simulink model "OneCombinedLQR"  (R2025b)
settings: Solver=ode4  StartTime=0.0  StopTime=T_end  FixedStep=0.001  RelTol=1e-3
values from neighbouring files (symbols this model uses):
  h_ref = double(h_ref)    [main.m]
  K_lqr = double(K_lqr)    [main.m]
  P = [x_ref y_ref]    [main.m]
  S_path = [S_path; S_raw(end)]    [main.m]
  theta_ref_unwrapped = unwrap(theta_ref)    [main.m]
  vd_path = min(vd_path, vd_max)    [main.m]
  wd_path = max(min(wd_path, wd_max), -wd_max)    [main.m]
  x_init = [phi_h; 0; theta_h; 0; v_h; omega_h; x_h; y_h]    [main.m]
settings Model: Creator=mwali  LastModifiedBy=mwali

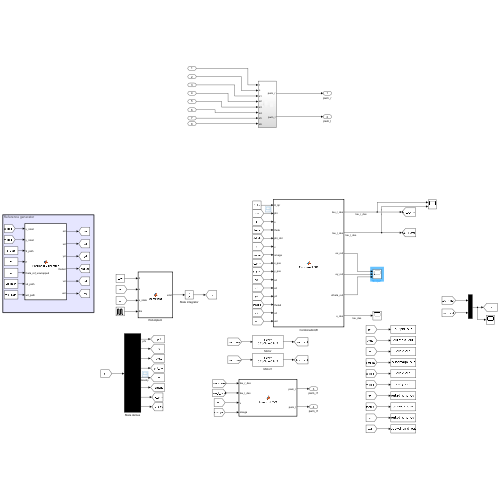
[thumbnail: Simulink's stored preview of the top-level diagram]
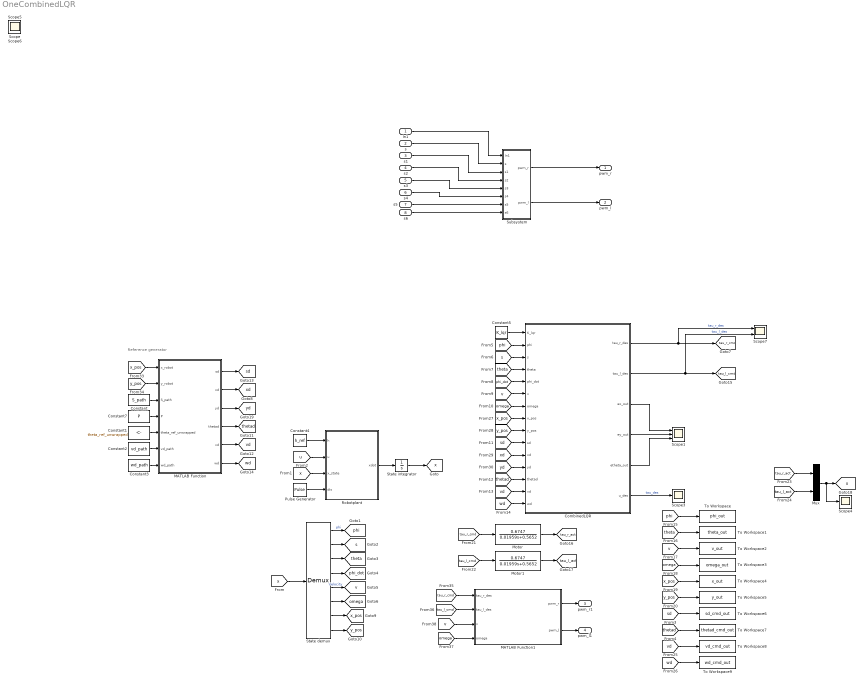
== system OneCombinedLQR ==
  note: Reference generator
  In1 : Inport
  s : Inport  Port=2
  s1 : Inport  Port=3
  s2 : Inport  Port=4
  s3 : Inport  Port=5
  s4 : Inport  Port=6
  s5 : Inport  Port=7
  s6 : Inport  Port=8
  CombinedLQR : MATLAB Function  TreatAsAtomicUnit=on
  Constant : Constant  Value=S_path
  Constant1 : Constant  Value=theta_ref_unwrapped
  Constant2 : Constant  Value=vd_path
  Constant3 : Constant  Value=wd_path
  Constant4 : Constant  Value=h_ref
  Constant5 : Constant  Value=K_lqr
  Constant7 : Constant  Value=P
  MATLAB Function : MATLAB Function  TreatAsAtomicUnit=on
  MATLAB Function1 : MATLAB Function  TreatAsAtomicUnit=on
  Motor : TransferFcn  Numerator=[0.6747]  Denominator=[0.01959 0.5652]
  Motor1 : TransferFcn  Numerator=[0.6747]  Denominator=[0.01959 0.5652]
  Mux : Mux  Inputs=2
  Pulse Generator : DiscretePulseGenerator  PulseType=Time based  Amplitude=0  Period=100  PhaseDelay=20
  Robotplant : MATLAB Function  TreatAsAtomicUnit=on
  Scope1 : Scope  NumInputPorts=3
      settings: ActiveDisplayYMinimum=-0.79993855795822744  ActiveDisplayYMaximum=1.6875243546714267  YLabel=distance [m]
  Scope{,3..6} (5 alike) : Scope
      Scope3 settings: ActiveDisplayYMinimum=-1.6865404665079047  ActiveDisplayYMaximum=1.5993577748502286  DataLoggingVariableName=ScopeData3
      Scope4 settings: ActiveDisplayYMinimum=-1  ActiveDisplayYMaximum=1  DataLoggingVariableName=ScopeData4
      Scope settings: ActiveDisplayYMinimum=-0.34848844243079913  ActiveDisplayYMaximum=2.6945477005962535
      Scope5 settings: ActiveDisplayYMinimum=-1  ActiveDisplayYMaximum=1  YLabel=angle[rad]  DataLoggingVariableName=ScopeData5
      Scope6 settings: ActiveDisplayYMinimum=-0.038382462899726216  ActiveDisplayYMaximum=0.22114533918550355  DataLoggingVariableName=ScopeData6
  Scope7 : Scope  NumInputPorts=2
      settings: ActiveDisplayYMinimum=-0.065744027020605431  ActiveDisplayYMaximum=0.033980624825214328  YLabel=torque[N.m]  DataLoggingVariableName=ScopeData7
  State demux : Demux  Outputs=8
  State integrator : Integrator  InitialCondition=x_init
  Subsystem : Subsystem
  To Workspace : ToWorkspace  VariableName=phi_out  SampleTime=-1
  To Workspace1 : ToWorkspace  VariableName=theta_out  SampleTime=-1
  To Workspace2 : ToWorkspace  VariableName=v_out  SampleTime=-1
  To Workspace3 : ToWorkspace  VariableName=omega_out  SampleTime=-1
  To Workspace4 : ToWorkspace  VariableName=x_out  SampleTime=-1
  To Workspace5 : ToWorkspace  VariableName=y_out  SampleTime=-1
  To Workspace6 : ToWorkspace  VariableName=sd_cmd_out  SampleTime=-1
  To Workspace7 : ToWorkspace  VariableName=thetad_cmd_out  SampleTime=-1
  To Workspace8 : ToWorkspace  VariableName=vd_cmd_out  SampleTime=-1
  To Workspace9 : ToWorkspace  VariableName=wd_cmd_out  SampleTime=-1
  pwm_r : Outport
  pwm_l : Outport  Port=2
  pwm_r1 : Outport  Port=3
  pwm_l1 : Outport  Port=4
  tag scope: omega=global, phi=global, phi_dot=global, s=global, sd=global, tau_l_act=global, tau_l_cmd=global, tau_r_act=global, tau_r_cmd=global, theta=global, thetad=global, u=global, v=global, vd=global, wd=global, x=global, x_pos=global, xd=global, y_pos=global, yd=global
  wires:
  In1/1 -> Subsystem/1(In1)
  s/1 -> Subsystem/2(s)
  s1/1 -> Subsystem/3(s1)
  s2/1 -> Subsystem/4(s2)
  s3/1 -> Subsystem/5(s3)
  s4/1 -> Subsystem/6(s4)
  s5/1 -> Subsystem/7(s5)
  s6/1 -> Subsystem/8(s6)
  Subsystem/1(pwm_r) -> pwm_r/1
  Subsystem/2(pwm_l) -> pwm_l/1
  [v] -> To Workspace2/1
  MATLAB Function1/2(pwm_l) -> pwm_l1/1
  [u] -> Robotplant/2(u)
  [s] -> CombinedLQR/3(s)
  MATLAB Function1/1(pwm_r) -> pwm_r1/1
  [vd] -> To Workspace8/1
  [theta] -> To Workspace1/1
  State demux/8 -> [y_pos]
  [x] -> Robotplant/3(x_state)
  [tau_r_cmd] -> MATLAB Function1/1(tau_r_des)
  [tau_l_act] -> Mux/2
  CombinedLQR/5(etheta_out) -> Scope1/3
  [phi] -> To Workspace/1
  [sd] -> CombinedLQR/10(sd)
  [tau_r_act] -> Mux/1
  Pulse Generator/1 -> Robotplant/4(dis)
  CombinedLQR/6(u_des) -> Scope3/1  "tau_des"
  [omega] -> To Workspace3/1
  [xd] -> CombinedLQR/11(xd)
  [yd] -> CombinedLQR/12(yd)
  CombinedLQR/1(tau_r_des) -> Scope7/1, [tau_r_cmd]  "tau_r_des"
  State demux/2 -> [s]
  [y_pos] -> CombinedLQR/9(y_pos)
  State demux/5 -> [v]  "Velocity"
  CombinedLQR/2(tau_l_des) -> Scope7/2, [tau_l_cmd]  "tau_l_des"
  MATLAB Function/4(thetad) -> [thetad]
  CombinedLQR/3(ex_out) -> Scope1/1
  State demux/6 -> [omega]
  [wd] -> CombinedLQR/15(wd)
  [omega] -> MATLAB Function1/4(omega)
  [v] -> CombinedLQR/6(v)
  [vd] -> CombinedLQR/14(vd)
  [y_pos] -> MATLAB Function/2(y_robot)
  State integrator/1 -> [x]
  [tau_l_cmd] -> MATLAB Function1/2(tau_l_des)
  [thetad] -> To Workspace7/1
  [phi_dot] -> CombinedLQR/5(phi_dot)
  Constant2/1 -> MATLAB Function/6(vd_path)
  Motor/1 -> [tau_r_act]
  Robotplant/1(xdot) -> State integrator/1
  MATLAB Function/3(yd) -> [yd]
  Constant5/1 -> CombinedLQR/1(K_lqr)
  State demux/7 -> [x_pos]
  [x_pos] -> CombinedLQR/8(x_pos)
  State demux/3 -> [theta]
  [wd] -> To Workspace9/1
  State demux/4 -> [phi_dot]
  MATLAB Function/6(wd) -> [wd]
  MATLAB Function/2(xd) -> [xd]
  [x_pos] -> To Workspace4/1
  [theta] -> CombinedLQR/4(theta)
  Constant4/1 -> Robotplant/1(h)
  Motor1/1 -> [tau_l_act]
  Mux/1 -> Scope4/1, [u]
  Constant7/1 -> MATLAB Function/4(P)
  [phi] -> CombinedLQR/2(phi)
  [tau_l_cmd] -> Motor1/1
  Constant/1 -> MATLAB Function/3(S_path)
  MATLAB Function/1(sd) -> [sd]
  CombinedLQR/4(ey_out) -> Scope1/2
  Constant3/1 -> MATLAB Function/7(wd_path)
  [omega] -> CombinedLQR/7(omega)
  [tau_r_cmd] -> Motor/1
  State demux/1 -> [phi]  "phi"
  Constant1/1 -> MATLAB Function/5(theta_ref_unwrapped)
  [thetad] -> CombinedLQR/13(thetad)
  [x] -> State demux/1
  [sd] -> To Workspace6/1
  MATLAB Function/5(vd) -> [vd]
  [y_pos] -> To Workspace5/1
  [x_pos] -> MATLAB Function/1(x_robot)
  [v] -> MATLAB Function1/3(v)

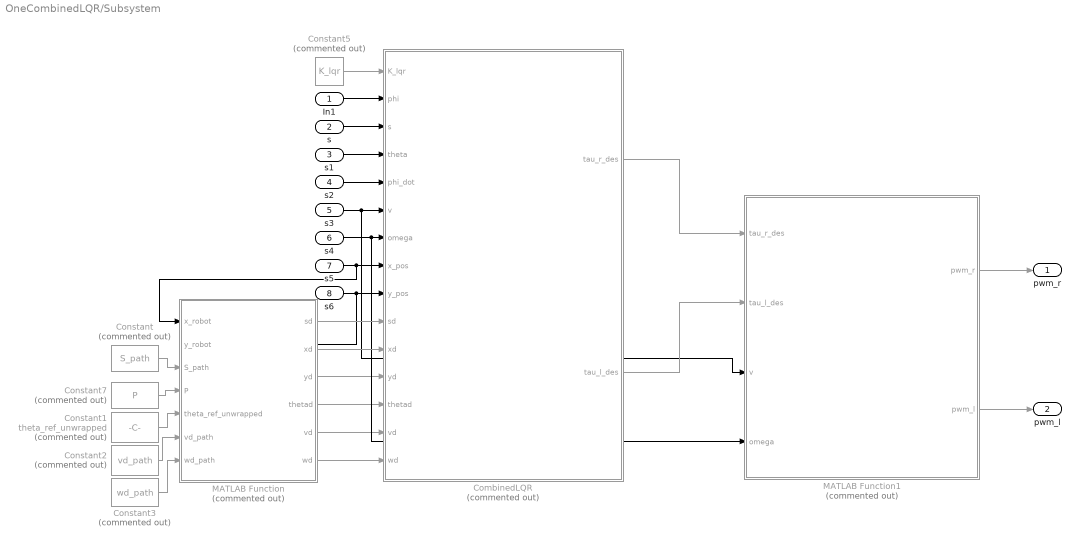
== system OneCombinedLQR/Subsystem ==
  In1 : Inport
  s : Inport  Port=2
  s1 : Inport  Port=3
  s2 : Inport  Port=4
  s3 : Inport  Port=5
  s4 : Inport  Port=6
  s5 : Inport  Port=7
  s6 : Inport  Port=8
  CombinedLQR : MATLAB Function  Commented=on  TreatAsAtomicUnit=on
  Constant : Constant  Commented=on  Value=S_path
  Constant1 : Constant  Commented=on  Value=theta_ref_unwrapped
  Constant2 : Constant  Commented=on  Value=vd_path
  Constant3 : Constant  Commented=on  Value=wd_path
  Constant5 : Constant  Commented=on  Value=K_lqr
  Constant7 : Constant  Commented=on  Value=P
  MATLAB Function : MATLAB Function  Commented=on  TreatAsAtomicUnit=on
  MATLAB Function1 : MATLAB Function  Commented=on  TreatAsAtomicUnit=on
  pwm_r : Outport
  pwm_l : Outport  Port=2
  wires:
  s3/1 -> MATLAB Function1/3(v), CombinedLQR/6(v)
  MATLAB Function1/2(pwm_l) -> pwm_l/1
  MATLAB Function/4(thetad) -> CombinedLQR/13(thetad)
  Constant3/1 -> MATLAB Function/7(wd_path)
  s5/1 -> MATLAB Function/1(x_robot), CombinedLQR/8(x_pos)
  s6/1 -> MATLAB Function/2(y_robot), CombinedLQR/9(y_pos)
  In1/1 -> CombinedLQR/2(phi)
  MATLAB Function/6(wd) -> CombinedLQR/15(wd)
  CombinedLQR/1(tau_r_des) -> MATLAB Function1/1(tau_r_des)
  MATLAB Function1/1(pwm_r) -> pwm_r/1
  MATLAB Function/5(vd) -> CombinedLQR/14(vd)
  CombinedLQR/2(tau_l_des) -> MATLAB Function1/2(tau_l_des)
  s2/1 -> CombinedLQR/5(phi_dot)
  Constant1/1 -> MATLAB Function/5(theta_ref_unwrapped)
  MATLAB Function/3(yd) -> CombinedLQR/12(yd)
  s4/1 -> MATLAB Function1/4(omega), CombinedLQR/7(omega)
  Constant7/1 -> MATLAB Function/4(P)
  Constant/1 -> MATLAB Function/3(S_path)
  MATLAB Function/2(xd) -> CombinedLQR/11(xd)
  Constant5/1 -> CombinedLQR/1(K_lqr)
  MATLAB Function/1(sd) -> CombinedLQR/10(sd)
  Constant2/1 -> MATLAB Function/6(vd_path)
  s1/1 -> CombinedLQR/4(theta)
  s/1 -> CombinedLQR/3(s)

== matlab function OneCombinedLQR/MATLAB Function ==
  data: x_robot input; y_robot input; S_path input; P input; theta_ref_unwrapped input; vd_path input; wd_path input; sd output; xd output; yd output; thetad output; vd output; wd output
function [sd, xd, yd, thetad, vd, wd] = ReferenceGenerator(x_robot, y_robot, S_path, P, theta_ref_unwrapped, vd_path, wd_path)
    N = size(P, 1);

    % 1. Find the nearest discrete node
    min_dist2 = inf;
    k_min = int32(1);
    for k = int32(1) : int32(N)
        dx = P(k, 1) - x_robot;
        dy = P(k, 2) - y_robot;
        d2 = dx*dx + dy*dy;
        if d2 < min_dist2
            min_dist2 = d2;
            k_min = k;
        end
    end

    % 2. Continuous Projection (Fixes the high-frequency torque chattering)
    k_next = min(k_min + int32(1), int32(N));
    k_prev = max(k_min - int32(1), int32(1));

    d2_next = (P(k_next,1)-x_robot)^2 + (P(k_next,2)-y_robot)^2;
    d2_prev = (P(k_prev,1)-x_robot)^2 + (P(k_prev,2)-y_robot)^2;

    if d2_next < d2_prev
        k1 = k_min;
        k2 = k_next;
    else
        k1 = k_prev;
        k2 = k_min;
    end

    if k1 == k2
        alpha = 0.0;
    else
        vx = P(k2,1) - P(k1,1);
        vy = P(k2,2) - P(k1,2);
        L2 = vx*vx + vy*vy;
        if L2 > 1e-6
            rx = x_robot - P(k1,1);
            ry = y_robot - P(k1,2);
            % Orthogonal projection scalar
            alpha = (rx*vx + ry*vy) / L2;
            alpha = max(0.0, min(1.0, alpha));
        else
            alpha = 0.0;
        end
    end

    % 3. Interpolate perfectly smooth references (No Lookahead)
    sd     = (1 - alpha) * S_path(k1) + alpha * S_path(k2);
    xd     = (1 - alpha) * P(k1, 1)   + alpha * P(k2, 1);
    yd     = (1 - alpha) * P(k1, 2)   + alpha * P(k2, 2);
    thetad = (1 - alpha) * theta_ref_unwrapped(k1) + alpha * theta_ref_unwrapped(k2);
    vd     = (1 - alpha) * vd_path(k1) + alpha * vd_path(k2);
    wd     = (1 - alpha) * wd_path(k1) + alpha * wd_path(k2);

    % 4. Safety clamps
    vd_max = 0.3;
    wd_max = 0.334;
    vd = max(0, min(vd, vd_max));
    wd = max(min(wd, wd_max), -wd_max);
end

== matlab function OneCombinedLQR/MATLAB Function1 ==
  data: tau_r_des input; pwm_r output; tau_l_des input; v input; omega input; pwm_l output
function [pwm_r, pwm_l] = TorqueToPWM(tau_r_des, tau_l_des, v, omega)
    % --- NFP-42GP-775-EN Motor Parameters ---
    K_t = 0.6746;      % Torque constant (Nm/A)
    K_e = 0.6746;      % Back-EMF constant (V/(rad/s))
    R_res = 0.9796;    % Armature resistance (Ohms)
    V_batt = 24.0;     % Battery voltage (V)
    
    % --- Controller & Robot Parameters ---
    max_pwm = 255;     % Change this if using a 10-bit or 12-bit timer!
    r = 0.060;         % Wheel radius (m)
    d = 0.450;         % Wheelbase/Track width (m)

    % 1. Estimate individual wheel rotational speeds (rad/s)
    omega_wheel_r = (v + (omega * d / 2)) / r;
    omega_wheel_l = (v - (omega * d / 2)) / r;

    % 2. Calculate right wheel PWM
    i_r = tau_r_des / K_t;
    v_r = (i_r * R_res) + (K_e * omega_wheel_r);
    pwm_float_r = (v_r / V_batt) * max_pwm;

    % 3. Calculate left wheel PWM
    i_l = tau_l_des / K_t;
    v_l = (i_l * R_res) + (K_e * omega_wheel_l);
    pwm_float_l = (v_l / V_batt) * max_pwm;

    % 4. Round to integer and clamp to valid ranges
    pwm_r = round(pwm_float_r);
    pwm_l = round(pwm_float_l);

    if pwm_r > max_pwm
        pwm_r = max_pwm; 
    elseif pwm_r < -max_pwm
        pwm_r = -max_pwm; 
    end
    
    if pwm_l > max_pwm
        pwm_l = max_pwm; 
    elseif pwm_l < -max_pwm
        pwm_l = -max_pwm; 
    end
end

== matlab function OneCombinedLQR/Robotplant ==
  data: h input; u input; xdot output; x_state input; dis input
function xdot = robotPlant(h, u, x_state,dis)

xdot = zeros(8,1);

% ---- Physical constants ----
Mw = 0.150;
Mb = 11.3;
r  = 0.060;
d  = 0.450;
Iw = 0.0002757224;
g  = 9.81;

% ---- Height-dependent parameters ----
Lc = -0.4748*h^2 + 1.2434*h - 0.0286;   % CoM height above wheel axle
Iy =  1.4948*h^2 + 0.5774*h - 0.0053;
Iz = -0.5689*h^2 + 0.1583*h + 0.1236;

% ---- Inertia matrix entries ----
M11   = Mb*Lc^2 + Iy;
M12   = Mb*Lc;
M22   = Mb + 2*Mw + 2*Iw/r^2;
M33   = (d^2/2)*Mw + (d^2/(2*r^2))*Iw + Iz;
Delta = M11*M22 - M12^2;

% Numerical safety
if abs(Delta) < 1e-8;  Delta = sign(Delta+1e-10)*1e-8; end
if abs(M33)   < 1e-8;  M33   = 1e-8; end

% ---- Unpack state ----
phi     = x_state(1);
% s     = x_state(2);   % not needed for dynamics
% theta = x_state(3);   % not needed for dynamics
phi_dot = x_state(4);
v       = x_state(5);
% omega = x_state(6);   % not needed for dynamics
theta_now = x_state(3);

% ---- Control inputs ----
tau_r = u(1);   % right-wheel torque [N*m]
tau_l = u(2);   % left-wheel torque  [N*m]

tau_sum  = tau_r + tau_l;
tau_diff = tau_r - tau_l;

% ---- Nonlinear generalized forces ----
% (derived from Lagrangian; see e.g. Grasser et al. 2002)
F_phi  = -M12 / (r * Delta) * tau_sum;           % torque -> phi_ddot channel
F_v    =  M11 / (r * Delta) * tau_sum;           % torque -> v_dot channel
F_yaw  =  d   / (2 * r * M33) * tau_diff;        % torque -> omega_dot channel

gravity_phi = (M22 * Mb * g * Lc) / Delta;       % phi channel gravity term
gravity_v   = (-M12 * Mb * g * Lc) / Delta;      % v channel gravity term
C_air = 2.5; 
wind_disturbance = -C_air * v * abs(v); 

% ---- FIX #1: nonlinear gravity term uses sin(phi) not phi ---- 
% Add the wind_disturbance to the pitch dynamics
phi_ddot  = gravity_phi * sin(phi) + F_phi + wind_disturbance - dis;
v_dot     = gravity_v   * sin(phi) + F_v;
omega_dot = F_yaw;

% ---- Kinematics ----
x_pos_dot = v * cos(theta_now);
y_pos_dot = v * sin(theta_now);

% ---- Assemble xdot ----
% [phi; s; theta; phi_dot; v; omega; x_pos; y_pos]
xdot(1) = phi_dot;        % d(phi)/dt
xdot(2) = v;              % d(s)/dt   = forward speed
xdot(3) = x_state(6);    % d(theta)/dt = omega
xdot(4) = phi_ddot;       % d(phi_dot)/dt  -- FIX #1
xdot(5) = v_dot;          % d(v)/dt        -- FIX #1
xdot(6) = omega_dot;      % d(omega)/dt
xdot(7) = x_pos_dot;      % d(x_pos)/dt
xdot(8) = y_pos_dot;      % d(y_pos)/dt

== matlab function OneCombinedLQR/Subsystem/CombinedLQR ==
  settings: updateMethod=DISCRETE
  data: K_lqr input; phi input; s input; theta input; phi_dot input; v input; omega input; x_pos input; y_pos input; sd input; xd input; yd input; thetad input; vd input; wd input; tau_r_des output; tau_l_des output
function [tau_r_des, tau_l_des] = CombinedLQR( ...
    K_lqr, phi, s, theta, phi_dot, v, omega, x_pos, y_pos, ...
    sd, xd, yd, thetad, vd, wd)
%#codegen

% outputs init
tau_r_des  = 0;
tau_l_des  = 0;
ex_out     = 0;
ey_out     = 0;
etheta_out = 0;

% -----------------------------
% 1) Path position error in world frame
% -----------------------------
dx = xd - x_pos;
dy = yd - y_pos;

% -----------------------------
% 2) Error in robot body frame
% ex = forward error
% et = lateral error
% -----------------------------
ex =  cos(theta)*dx + sin(theta)*dy;
ey = -sin(theta)*dx + cos(theta)*dy;

% save for plotting
ex_out = ex;
ey_out = ey;

% -----------------------------
% 3) Heading correction from lateral error
% -----------------------------
k_y = 0.1;                     % tune this if needed
theta_corr_max = deg2rad(20);  % max heading correction

theta_corr = k_y * ey;

if theta_corr > theta_corr_max
    theta_corr = theta_corr_max;
elseif theta_corr < -theta_corr_max
    theta_corr = -theta_corr_max;
end

thetad_corr = thetad + theta_corr;

% -----------------------------
% 4) State error for LQR
% -----------------------------
e = zeros(6,1);
e(1) =phi ;
e(2) = s - sd; 
e(3) = atan2(sin(theta - thetad_corr), cos(theta - thetad_corr));
e(4) = phi_dot;
e(5) = v - vd;
e(6) = omega - wd;

etheta_out = e(3);

% -----------------------------
% 5) LQR control
% -----------------------------
u_des = -K_lqr * e;

tau_r_des = u_des(1);
tau_l_des = u_des(2);

% -----------------------------
% 6) Torque saturation
% -----------------------------
tau_lim = 3; % Changed from 6 to 3

if tau_r_des > tau_lim
    tau_r_des = tau_lim;
elseif tau_r_des < -tau_lim
    tau_r_des = -tau_lim;
end

if tau_l_des > tau_lim
    tau_l_des = tau_lim;
elseif tau_l_des < -tau_lim
    tau_l_des = -tau_lim;
end

== matlab function OneCombinedLQR/Subsystem/MATLAB Function ==
  data: x_robot input; y_robot input; S_path input; P input; theta_ref_unwrapped input; vd_path input; wd_path input; sd output; xd output; yd output; thetad output; vd output; wd output
function [sd, xd, yd, thetad, vd, wd] = ReferenceGenerator(x_robot, y_robot, S_path, P, theta_ref_unwrapped, vd_path, wd_path)
    N = size(P, 1);

    % 1. Find the nearest discrete node
    min_dist2 = inf;
    k_min = int32(1);
    for k = int32(1) : int32(N)
        dx = P(k, 1) - x_robot;
        dy = P(k, 2) - y_robot;
        d2 = dx*dx + dy*dy;
        if d2 < min_dist2
            min_dist2 = d2;
            k_min = k;
        end
    end

    % 2. Continuous Projection (Fixes the high-frequency torque chattering)
    k_next = min(k_min + int32(1), int32(N));
    k_prev = max(k_min - int32(1), int32(1));

    d2_next = (P(k_next,1)-x_robot)^2 + (P(k_next,2)-y_robot)^2;
    d2_prev = (P(k_prev,1)-x_robot)^2 + (P(k_prev,2)-y_robot)^2;

    if d2_next < d2_prev
        k1 = k_min;
        k2 = k_next;
    else
        k1 = k_prev;
        k2 = k_min;
    end

    if k1 == k2
        alpha = 0.0;
    else
        vx = P(k2,1) - P(k1,1);
        vy = P(k2,2) - P(k1,2);
        L2 = vx*vx + vy*vy;
        if L2 > 1e-6
            rx = x_robot - P(k1,1);
            ry = y_robot - P(k1,2);
            % Orthogonal projection scalar
            alpha = (rx*vx + ry*vy) / L2;
            alpha = max(0.0, min(1.0, alpha));
        else
            alpha = 0.0;
        end
    end

    % 3. Interpolate perfectly smooth references (No Lookahead)
    sd     = (1 - alpha) * S_path(k1) + alpha * S_path(k2);
    xd     = (1 - alpha) * P(k1, 1)   + alpha * P(k2, 1);
    yd     = (1 - alpha) * P(k1, 2)   + alpha * P(k2, 2);
    thetad = (1 - alpha) * theta_ref_unwrapped(k1) + alpha * theta_ref_unwrapped(k2);
    vd     = (1 - alpha) * vd_path(k1) + alpha * vd_path(k2);
    wd     = (1 - alpha) * wd_path(k1) + alpha * wd_path(k2);

    % 4. Safety clamps
    vd_max = 0.3;
    wd_max = 0.334;
    vd = max(0, min(vd, vd_max));
    wd = max(min(wd, wd_max), -wd_max);
end

== matlab function OneCombinedLQR/CombinedLQR ==
  settings: updateMethod=DISCRETE
  data: K_lqr input; phi input; s input; theta input; phi_dot input; v input; omega input; x_pos input; y_pos input; sd input; xd input; yd input; thetad input; vd input; wd input; tau_r_des output; tau_l_des output; ex_out output; ey_out output; etheta_out output; u_des output
function [tau_r_des, tau_l_des, ex_out, ey_out, etheta_out, u_des] = CombinedLQR( ...
    K_lqr, phi, s, theta, phi_dot, v, omega, x_pos, y_pos, ...
    sd, xd, yd, thetad, vd, wd)
%#codegen

% outputs init
tau_r_des  = 0;
tau_l_des  = 0;
ex_out     = 0;
ey_out     = 0;
etheta_out = 0;

% -----------------------------
% 1) Path position error in world frame
% -----------------------------
dx = xd - x_pos;
dy = yd - y_pos;

% -----------------------------
% 2) Error in robot body frame
% ex = forward error
% et = lateral error
% -----------------------------
ex =  cos(theta)*dx + sin(theta)*dy;
ey = -sin(theta)*dx + cos(theta)*dy;

% save for plotting
ex_out = ex;
ey_out = ey;

% -----------------------------
% 3) Heading correction from lateral error
% -----------------------------
k_y = 0.1;                     % tune this if needed
theta_corr_max = deg2rad(20);  % max heading correction

theta_corr = k_y * ey;

if theta_corr > theta_corr_max
    theta_corr = theta_corr_max;
elseif theta_corr < -theta_corr_max
    theta_corr = -theta_corr_max;
end

thetad_corr = thetad + theta_corr;

% -----------------------------
% 4) State error for LQR
% -----------------------------
e = zeros(6,1);
e(1) =phi ;
e(2) = s - sd; 
e(3) = atan2(sin(theta - thetad_corr), cos(theta - thetad_corr));
e(4) = phi_dot;
e(5) = v - vd;
e(6) = omega - wd;

etheta_out = e(3);

% -----------------------------
% 5) LQR control
% -----------------------------
u_des = -K_lqr * e;

tau_r_des = u_des(1);
tau_l_des = u_des(2);

% -----------------------------
% 6) Torque saturation
% -----------------------------
tau_lim = 3; % Changed from 6 to 3

if tau_r_des > tau_lim
    tau_r_des = tau_lim;
elseif tau_r_des < -tau_lim
    tau_r_des = -tau_lim;
end

if tau_l_des > tau_lim
    tau_l_des = tau_lim;
elseif tau_l_des < -tau_lim
    tau_l_des = -tau_lim;
end

== matlab function OneCombinedLQR/Subsystem/MATLAB Function1 ==
  data: tau_r_des input; pwm_r output; tau_l_des input; v input; omega input; pwm_l output
function [pwm_r, pwm_l] = TorqueToPWM(tau_r_des, tau_l_des, v, omega)
    % --- NFP-42GP-775-EN Motor Parameters ---
    K_t = 0.6746;      % Torque constant (Nm/A)
    K_e = 0.6746;      % Back-EMF constant (V/(rad/s))
    R_res = 0.9796;    % Armature resistance (Ohms)
    V_batt = 24.0;     % Battery voltage (V)
    
    % --- Controller & Robot Parameters ---
    max_pwm = 255;     % Change this if using a 10-bit or 12-bit timer!
    r = 0.060;         % Wheel radius (m)
    d = 0.450;         % Wheelbase/Track width (m)

    % 1. Estimate individual wheel rotational speeds (rad/s)
    omega_wheel_r = (v + (omega * d / 2)) / r;
    omega_wheel_l = (v - (omega * d / 2)) / r;

    % 2. Calculate right wheel PWM
    i_r = tau_r_des / K_t;
    v_r = (i_r * R_res) + (K_e * omega_wheel_r);
    pwm_float_r = (v_r / V_batt) * max_pwm;

    % 3. Calculate left wheel PWM
    i_l = tau_l_des / K_t;
    v_l = (i_l * R_res) + (K_e * omega_wheel_l);
    pwm_float_l = (v_l / V_batt) * max_pwm;

    % 4. Round to integer and clamp to valid ranges
    pwm_r = round(pwm_float_r);
    pwm_l = round(pwm_float_l);

    if pwm_r > max_pwm
        pwm_r = max_pwm; 
    elseif pwm_r < -max_pwm
        pwm_r = -max_pwm; 
    end
    
    if pwm_l > max_pwm
        pwm_l = max_pwm; 
    elseif pwm_l < -max_pwm
        pwm_l = -max_pwm; 
    end
end
